simulink model "Two_DPSK"  (R2013a)
settings: Solver=ode45  StartTime=0.0  StopTime=10.0  RelTol=1e-3
libraries: dsparch4 x2, commrandsrc2 x2, commnoisgen2 x1, commsrccod2 x1, commutil2 x1
settings Model: Creator=sliencer  LastModifiedBy=sliencer

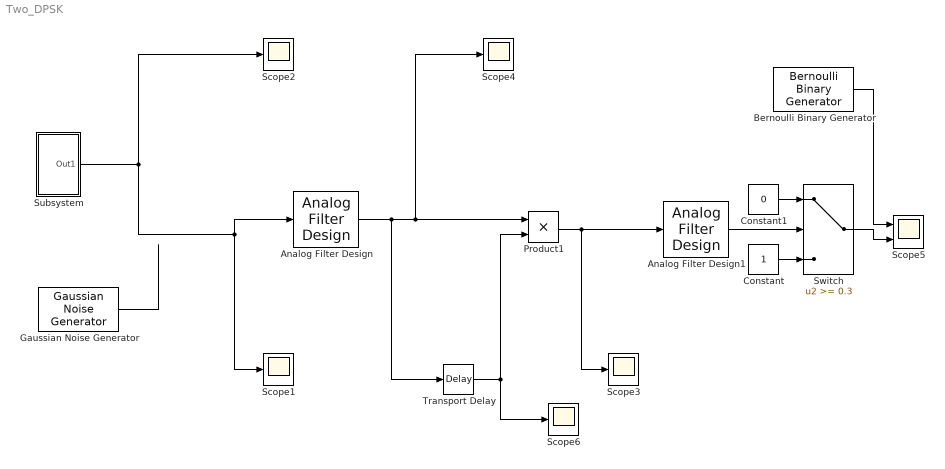
== system Two_DPSK ==
  Analog Filter Design : dsparch4/Analog Filter Design  method=Butterworth  filttype=Bandpass  N=4  Wlo=2*2*pi  Whi=7*2*pi  Rp=2  Rs=40
  Analog Filter Design1 : dsparch4/Analog Filter Design  method=Butterworth  filttype=Lowpass  N=4  Wlo=3*2*pi  Whi=80  Rp=2  Rs=40
  Bernoulli Binary Generator : commrandsrc2/Bernoulli Binary Generator  P=0.5  seed=61  Ts=1  frameBased=off  sampPerFrame=1  orient=off  outDataType=double
  Constant : Constant
  Constant1 : Constant  Value=0
  Gaussian Noise Generator : commnoisgen2/Gaussian Noise Generator  m=0  d=1  s=41  Ts=1  frameBased=off  sampPerFrame=1  orient=off  outDataType=double
  Product1 : Product
  Scope{1..4,6} (5 alike) : Scope
      Scope2 settings: SaveName=ScopeData2
      Scope3 settings: SaveName=ScopeData3
      Scope4 settings: SaveName=ScopeData4
      Scope6 settings: SaveName=ScopeData6
  Scope5 : Scope  NumInputPorts=2
      settings: YMin=-5~-5  YMax=5~5  SaveName=ScopeData5
  Subsystem : Subsystem
  Switch : Switch  Threshold=0.3
  Transport Delay : TransportDelay  DelayTime=0.318*pi
  wires:
  Gaussian Noise Generator/1 -> ?
  Subsystem/1(Out1) -> Analog Filter Design/1, Scope1/1, Scope2/1
  Analog Filter Design/1 -> Transport Delay/1, Scope4/1, Product1/1
  Transport Delay/1 -> Scope6/1, Product1/2
  Product1/1 -> Scope3/1, Analog Filter Design1/1
  Analog Filter Design1/1 -> Switch/2
  Switch/1 -> Scope5/2
  Bernoulli Binary Generator/1 -> Scope5/1
  Constant/1 -> Switch/3
  Constant1/1 -> Switch/1

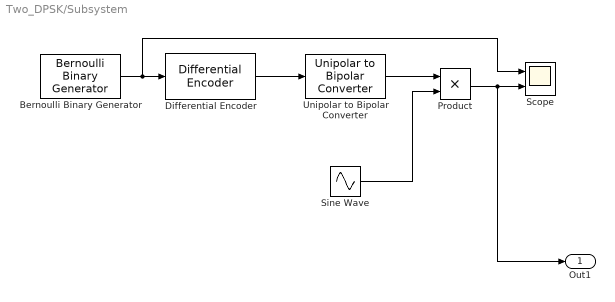
== system Two_DPSK/Subsystem ==
  Bernoulli Binary Generator : commrandsrc2/Bernoulli Binary Generator  P=0.5  seed=61  Ts=1  frameBased=off  sampPerFrame=1  orient=off  outDataType=double
  Differential Encoder : commsrccod2/Differential Encoder  InitCond=0.05
  Product : Product
  Scope : Scope  NumInputPorts=2
      settings: YMin=-5~-5  YMax=5~5
  Sine Wave : Sin  Frequency=8*pi  SampleTime=1/500
  Unipolar to Bipolar Converter : commutil2/Unipolar to Bipolar Converter  M=2  polarity=Positive  dataType=Same as input
  Out1 : Outport
  wires:
  Differential Encoder/1 -> Unipolar to Bipolar Converter/1
  Unipolar to Bipolar Converter/1 -> Product/1
  Sine Wave/1 -> Product/2
  Product/1 -> Scope/2, Out1/1
  Bernoulli Binary Generator/1 -> Scope/1, Differential Encoder/1
